simulink model "GradientAscentTrialTesting"  (R2017b)
settings: Solver=FixedStepDiscrete  StartTime=0.0  StopTime=60  FixedStep=Ts  RelTol=1e-3
PreLoadFcn:
  | ROSconfig
  | wptsSignalSetup
InitFcn:
  | config_parameters
StartFcn:
  | gazeboSetup
StopFcn:
  | gazeboReset
  | goalreset
  | loadResults
model workspace (MAT data in the model file):
  goalpoints = Simulink.Signal
  goalpoints.DataType = 'auto'
  goalpoints.Dimensions = -1
  goalpoints.DimensionsMode = 'auto'
  goalpoints.Complexity = 'auto'
  goalpoints.SampleTime = -1
  goalpoints.SamplingMode = 'auto'
  goals = Simulink.Signal
  goals.DataType = 'auto'
  goals.Dimensions = -1
  goals.DimensionsMode = 'auto'
  goals.Complexity = 'auto'
  goals.SampleTime = -1
  goals.SamplingMode = 'auto'
  idx = 1
  y = Simulink.Parameter
  y.DataType = 'auto'
  y.Dimensions = [0 0]
values from neighbouring files (symbols this model uses):
  m = [m; i*(2*pi/M)]    [SensorArrangementPlots.m]    (also in sensorArrayTesting.m = [0;0;1.2566;2.5133;3.7699;5.0265])
  sensorDist = 1    [GradientAscentMetrics.m]
undefined symbols (not defined in the file or in its folder): angmax, Angular, concDetectionAccuracy, Cthresh, DiscIntNeverNeededParam, distError, dynamicPlume, hot, inc, init, initX, initY, Kd, Ki, Kp, Linear, N, Offset, PlumeD, PlumeUpdateRate, Res, sourceAccuracy, T, Ts, vmax, wgain, WindD, WindX, x_g, y_g
libraries: simulink x21, dspindex x18, dspswit3 x4, robotlib x3, sm_lib x2, nesl_utility x1, dspsnks4 x1, mobileRoboticsLib x1
(part 1 of 2)
PauseFcn:
  | gazeboPause
settings Model: OrderedModelArguments=off  Creator=ty  LastModifiedBy=ty
settings SolverCC: AlgebraicLoopSolver=LineSearch
settings DataIOCC: ExternalInput=[r, b]  SaveFormat=Array  SaveState=on  InspectSignalLogs=on  StateSaveName=wpts
settings SimMechanicsCC: VisOnUpdateDiagram=on  VisDuringSimulation=on  DefaultBodyColor=[.877 0 0]
settings ExplorerConfigSet: SimMechanicsOpenEditorOnUpdate=off  InternalSimMechanicsExplorerSettings="<ExplorerConfiguration><canonicalview>default</canonicalview><AnimationSetting><BasePlaybackSpeed>1.0</BasePlaybackSpeed><PlaybackSpeedFactor>4.0</PlaybackSpeedFactor></AnimationSetting><TilePanel><TileInfo><Tiles Columns=\"2\" Count=\"4\" Rows=\"2\"><Column Weight=\"0.5\"/><Column Weight=\"0.5\"/><Row Weight=\"0.5\"/><Row Weight=\"0.5\"/><Tile Height=\"1\" Width=\"1\" X=\"0\" Y=\"0\"/><Tile Height=\"1\" Width=\"1\" X=\"0\" Y=\"1\"/><Tile Height=\"1\" Width=\"1\" X=\"1\" Y=\"0\"/><Tile Height=\"1\" Width=\"1\" X=\"1\" Y=\"1\"/></Tiles></TileInfo><SceneInfo><SceneViewer><BGColor><R>0.60000002384185791</R><G>0.60000002384185791</G><B>0.60000002384185791</B></BGColor><Camera><DoPerspective>off</DoPerspective><Position><X>0.523539858098702515</X><Y>-0.526832295844210763</Y><Z>1.31558763938248235</Z></Position><Center><X>0.523539858098702515</X><Y>-0.526832295844210763</Y><Z>0.315587639382482354</Z></Center><Up><X>0</X><Y>1</Y><Z>-0</Z></Up><ViewLimDist>1</ViewLimDist><YLim>8.09056691591361421</YLim><XLim>11.4549610789668002</XLim></Camera></SceneViewer><SceneViewer><BGColor><R>0.60000002384185791</R><G>0.60000002384185791</G><B>0.60000002384185791</B></BGColor><Camera><DoPerspective>off</DoPerspective><Position><X>-1.00000000034924597</X><Y>-0.123102183445061519</Y><Z>0.275798201199813964</Z></Position><Center><X>-3.49245965480804443e-10</X><Y>-0.123102183445061519</Y><Z>0.275798201199813964</Z></Center><Up><X>0</X><Y>0</Y><Z>1</Z></Up><ViewLimDist>1</ViewLimDist><YLim>3.47753295219900371</YLim><XLim>4.92363576400452985</XLim></Camera></SceneViewer><SceneViewer><BGColor><R>0.60000002384185791</R><G>0.60000002384185791</G><B>0.60000002384185791</B></BGColor><Camera><DoPerspective>off</DoPerspective><Position><X>0.692144908773628886</X><Y>-0.692774488443842151</Y><Z>0.641997243049143074</Z></Position><Center><X>0.114794639584003433</X><Y>-0.115424219254216046</Y><Z>0.0646469738595174259</Z></Center><Up><X>-0.408248290463863073</X><Y>0.408248290463863073</Y><Z>0.816496580927726145</Z></Up><ViewLimDist>1</ViewLimDist><YLim>6.0070720394774666</YLim><XLim>8.50506239252750262</XLim></Camera></SceneViewer><SceneViewer><BGColor><R>0.60000002384185791</R><G>0.60000002384185791</G><B>0.60000002384185791</B></BGColor><Camera><DoPerspective>off</DoPerspective><Position><X>0.0489598554332313918</X><Y>-0.287272213681231237</Y><Z>1.31558770067272501</Z></Position><Center><X>0.0489598554332313918</X><Y>-0.287272213681231237</Y><Z>0.315587700672725013</Z></Center><Up><X>0</X><Y>1</Y><Z>-0</Z></Up><ViewLimDist>1</ViewLimDist><YLim>2.42704539801906094</YLim><XLim>3.4363118011556999</XLim></Camera></SceneViewer></SceneInfo></TilePanel><MechEditorPanel><Cameras><Camera><Id>Camera1</Id><Value><Name>TopCamera1</Name><NativeCamera><PositionKeyframeSet><Keyframe><Time>+0.0000000000000000e+00</Time><Value><X>+2.1442706964244174e-01</X><Y>+2.3082412087368320e-01</Y><Z>+8.5801428178680403e+00</Z></Value></Keyframe></PositionKeyframeSet><CenterKeyframeSet><Keyframe><Time>+0.0000000000000000e+00</Time><Value><X>+1.7666087274208450e-01</X><Y>+1.6219238056249624e-01</Y><Z>+3.9566976367888529e-01</Z></Value></Keyframe></CenterKeyframeSet><UpVectorKeyframeSet><Keyframe><Time>+0.0000000000000000e+00</Time><Value><X>-1.4536948631457236e-02</X><Y>+9.9985973958876295e-01</Y><Z>-8.3173477730344968e-03</Z></Value></Keyframe></UpVectorKeyframeSet></NativeCamera></Value></Camera></Cameras><GfxPanelCameraMap/><VideoCreator><PlaybackSpeedRatio>1.0</PlaybackSpeedRatio><FrameRate>30</FrameRate><VideoFormat>Motion JPEG AVI</VideoFormat><FrameSize>auto</FrameSize></VideoCreator></MechEditorPanel></ExplorerConfiguration>"

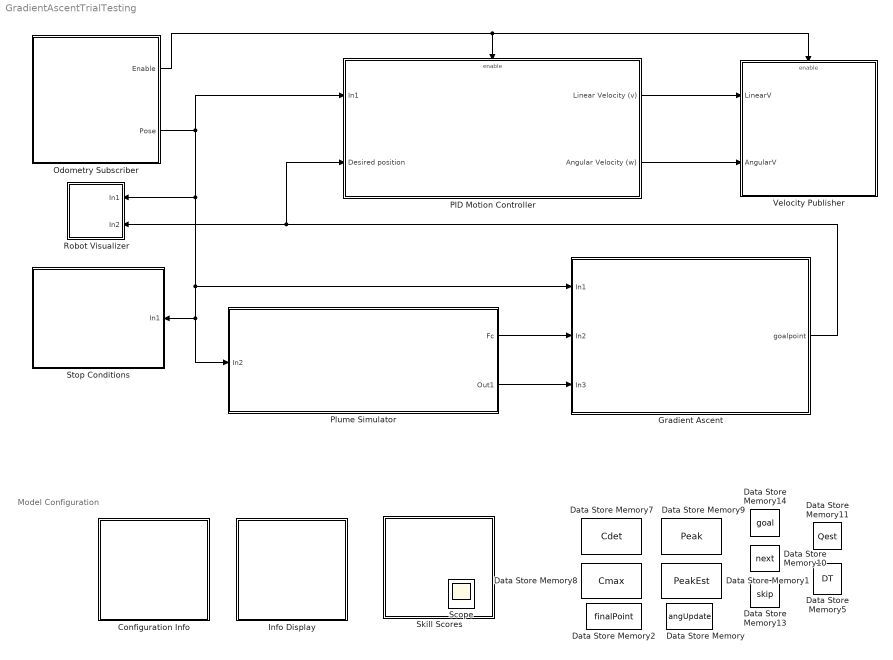
== system GradientAscentTrialTesting ==
  note: Model Configuration
  Configuration Info : Subsystem
  Data Store Memory : DataStoreMemory  DataStoreName=angUpdate  ReadBeforeWriteMsg=warning  WriteAfterWriteMsg=warning  WriteAfterReadMsg=warning  ShowAdditionalParam=off
  Data Store Memory1 : DataStoreMemory  DataStoreName=PeakEst  ReadBeforeWriteMsg=warning  WriteAfterWriteMsg=warning  WriteAfterReadMsg=warning  InitialValue=[(initX) (initY)]  VectorParams1D=off  ShowAdditionalParam=off
  Data Store Memory10 : DataStoreMemory  DataStoreName=next  ReadBeforeWriteMsg=warning  WriteAfterWriteMsg=warning  WriteAfterReadMsg=warning  ShowAdditionalParam=off
  Data Store Memory11 : DataStoreMemory  DataStoreName=Qest  ReadBeforeWriteMsg=warning  WriteAfterWriteMsg=warning  WriteAfterReadMsg=warning  ShowAdditionalParam=off
  Data Store Memory13 : DataStoreMemory  DataStoreName=skip  ReadBeforeWriteMsg=warning  WriteAfterWriteMsg=warning  WriteAfterReadMsg=warning  ShowAdditionalParam=off
  Data Store Memory14 : DataStoreMemory  DataStoreName=goal  ReadBeforeWriteMsg=warning  WriteAfterWriteMsg=warning  WriteAfterReadMsg=warning  VectorParams1D=off  ShowAdditionalParam=off
  Data Store Memory2 : DataStoreMemory  DataStoreName=finalPoint  ReadBeforeWriteMsg=warning  WriteAfterWriteMsg=warning  WriteAfterReadMsg=warning  ShowAdditionalParam=off
  Data Store Memory5 : DataStoreMemory  DataStoreName=DT  ReadBeforeWriteMsg=warning  WriteAfterWriteMsg=warning  WriteAfterReadMsg=warning  InitialValue=[0]  VectorParams1D=off  ShowAdditionalParam=off
  Data Store Memory7 : DataStoreMemory  DataStoreName=Cdet  ReadBeforeWriteMsg=warning  WriteAfterWriteMsg=warning  WriteAfterReadMsg=warning  ShowAdditionalParam=off
  Data Store Memory8 : DataStoreMemory  DataStoreName=Cmax  ReadBeforeWriteMsg=warning  WriteAfterWriteMsg=warning  WriteAfterReadMsg=warning  ShowAdditionalParam=off
  Data Store Memory9 : DataStoreMemory  DataStoreName=Peak  ReadBeforeWriteMsg=warning  WriteAfterWriteMsg=warning  WriteAfterReadMsg=warning  InitialValue=[x_g,y_g]  ShowAdditionalParam=off
  Gradient Ascent : Subsystem  mask{sensorDist=.5, mag=2}
      mask prompts: sensorDist "Sensor Distance"; mag "Update Magnitude"
  Info Display : Subsystem
  Odometry Subscriber : Subsystem
  PID Motion Controller : Subsystem
  Plume Simulator : Subsystem
  Robot Visualizer : Subsystem
  Skill Scores : Subsystem
  Stop Conditions : Subsystem
  Velocity Publisher : Subsystem
  Scope : Scope
  wires:
  Odometry Subscriber/1(Enable) -> Velocity Publisher/Enable, PID Motion Controller/Enable
  Odometry Subscriber/2(Pose) -> Plume Simulator/1(In2), Stop Conditions/1(In1), Gradient Ascent/1(In1), Robot Visualizer/1(In1), PID Motion Controller/1(In1)
  PID Motion Controller/1(Linear Velocity (v)) -> Velocity Publisher/1(LinearV)
  PID Motion Controller/2(Angular Velocity (w)) -> Velocity Publisher/2(AngularV)
  Gradient Ascent/1(goalpoint) -> PID Motion Controller/2(Desired position), Robot Visualizer/2(In2)
  Plume Simulator/1(Fc) -> Gradient Ascent/2(In2)
  Plume Simulator/2(Out1) -> Gradient Ascent/3(In3)

== system GradientAscentTrialTesting/Configuration Info ==
  note: Nodes :
      | Publishers:
      | /sim_p3at/cmd_vel
      | /toggle_led
      | Subscribers:
      | /sim_p3at/odom
      | Messages:
      | geometry_msgs/Twist
      | std_msgs/Empty
  note: Startup Programs :
      | roscore
      | roslaunch nre_p3at p3at.gazebo.launch (starts Gazebo and /sim_p3at Nodes)
      | Arduino: ledtest3.ino
      | rosrun rosserial_python serial_node.py /dev/ttyACM0
      | MATLAB: (Simulink project)
  note: SS Parameters :
      | Expansion Constant: 2
  note: Plume Parameters :
      |
      | Diffusion constant (m2/s): c_diff = .8
      |
      | Advection velocity values (m/s): ux = 0 uy = 0 uz = 0.2
      |
      | Simulation Time (seconds): T = 10
      |
      | Domain dimensions (meters): L = 50 B = 50 H = 5
  "Counter " : Subsystem  Commented=on
  Floating Scope : Scope  Commented=on
      settings: Floating=on
  MechanismConfiguration : sm_lib/Utilities/Mechanism Configuration  UniformGravity=Constant  GravityVector=[0 0 -9.80665]  GravityUnits=m/s^2  LinearizationDelta=0.01
  Solver Configuration : nesl_utility/Solver Configuration  PhysicalDomain=network_engine_domain  SubClassName=solver  LeftPortType=input  RightPortType=generic  Accelerate=off  Tones=[]  Harmonics=[]  SimulateNoise=off  Profile=off  UseLocalSampling=off  EnableSwitchedLinearOptims=on  FrequencyDomain=off  UseCCode=off  RelTol=0.001  AbsTol=1e-06  MinStep=1e-09  ToWorkspace=off  RevertToSquareIcSolve=off  NumHomotopyIterations=100  PhasorMode=off  PhasorModeNumHarmonics=1  DoDC=on  ResidualTolerance=1e-09  UseLocalSolver=on  LocalSolverChoice=NE_BACKWARD_EULER_ADVANCER  LocalSolverSampleTime=Ts  DoFixedCost=on  MaxNonlinIter=3  MaxModeIter=2  LinearAlgebra=Sparse  DelaysMemoryBudget=1024  AutomaticFiltering=on  FilteringTimeConstant=0.01
  World : sm_lib/Frames and Transforms/World Frame
  connections:
  MechanismConfiguration/RConn1 -- World/RConn1 -- Solver Configuration/RConn1

== system GradientAscentTrialTesting/Gradient Ascent ==
  In1 : Inport
  In2 : Inport  Port=2
  In3 : Inport  Port=3
  Constant : Constant  Value=sensorDist
  Constant1 : Constant  Value=N
  Data Store Read : DataStoreRead  DataStoreName=next
  Data Store Write : DataStoreWrite  DataStoreName=angUpdate
  Detect Change : simulink/Logic and Bit Operations/Detect Change  vinit=1.514  OutDataTypeStr=boolean
  Display : Display
  GradAscent : MATLAB Function  TreatAsAtomicUnit=on
  Subsystem1 : Subsystem
  goalpoint : Outport
  wires:
  In1/1 -> Subsystem1/1(pose)
  In2/1 -> GradAscent/1(C)
  In3/1 -> GradAscent/2(n)
  GradAscent/1(ang) -> Detect Change/1, Display/1, Subsystem1/3(ang)
  Subsystem1/1(goal) -> goalpoint/1
  Data Store Read/1 -> Subsystem1/2(next)
  Constant/1 -> GradAscent/4(r)
  Constant1/1 -> GradAscent/3(N)
  Detect Change/1 -> Data Store Write/1

== system GradientAscentTrialTesting/Info Display ==
  Clock : Clock
      settings: Decimation=2
  Data Store Read : DataStoreRead  DataStoreName=PeakEst
  Data Store Read1 : DataStoreRead  DataStoreName=Peak
  Data Store Read2 : DataStoreRead  DataStoreName=Cmax
  Data Store Read3 : DataStoreRead  DataStoreName=Cdet
  Data Store Read4 : DataStoreRead  DataStoreName=Qest
  Detected Concentration Levels : Subsystem  DialogController=hmiCreateDDGDialog  IsWebBlock=on  mask(MWDashboardBlock){webBlockId=6b377d99-0008-4121-aea7-73876731bd10, webBlockType=sdiscope, ShowInitialText=off, HMISrcModelName=GradientAscentTrialTesting}
      mask prompts: webBlockId "WebBlock Id"; webBlockType "WebBlock Type"; HMISrcModelName "Source Model"
      mask help: SimulinkHMI:dialogs:HMIScopeDialogDesc
      mask Help: helpview([docroot '/mapfiles/simulink.map'], 'hmi_scope')
      mask Display:
      | if strcmp(get_param(bdroot(gcb),'BlockDiagramType'), 'library')
      |     image([(matlabroot) '/toolbox/simulink/hmi/icons/DashboardScope.png']);
      | end
  Display{,1..5} (6 alike) : Display
  Localization Error : Subsystem  DialogController=hmiCreateDDGDialog  IsWebBlock=on  mask(MWDashboardBlock){webBlockId=d5e779f4-6058-4c24-8153-4ecbd3312a81, webBlockType=sdiscope, ShowInitialText=on, HMISrcModelName=GradientAscentTrialTesting}
      mask prompts: webBlockId "WebBlock Id"; webBlockType "WebBlock Type"; HMISrcModelName "Source Model"
      mask help: SimulinkHMI:dialogs:HMIScopeDialogDesc
      mask Help: helpview([docroot '/mapfiles/simulink.map'], 'hmi_scope')
      mask Display:
      | if strcmp(get_param(bdroot(gcb),'BlockDiagramType'), 'library')
      |     image([(matlabroot) '/toolbox/simulink/hmi/icons/DashboardScope.png']);
      | end
  To Workspace : ToWorkspace  VariableName=Tm  SampleTime=-1
  wires:
  Data Store Read1/1 -> Display/1
  Data Store Read/1 -> Display4/1
  Data Store Read4/1 -> Display3/1
  Data Store Read2/1 -> Display2/1
  Clock/1 -> To Workspace/1, Display1/1
  Data Store Read3/1 -> Display5/1

== system GradientAscentTrialTesting/Odometry Subscriber ==
  Odom Conversion : Subsystem
  Subscribe1 : robotlib/Subscribe  SourceLibraryInfo=This block requires Robotics System Toolbox  topicSource=Select from ROS network  topic=/sim_p3at/odom  messageType=nav_msgs/Odometry  sampleTime=-1  messageQueueLength=51
      settings: SourceProductBaseCode=RO
  Enable : Outport
  Pose : Outport  Port=2
  wires:
  Subscribe1/1 -> Enable/1
  Subscribe1/2 -> Odom Conversion/1(In1)
  Odom Conversion/1(pose) -> Pose/1

== system GradientAscentTrialTesting/PID Motion Controller ==
  In1 : Inport
  Desired position : Inport  Port=2
  Enable : EnablePort
  Constant3 : Constant  Value=0
  Demux : Demux  Outputs=3
  PID Calculations : Subsystem  mask{distThresh=0.5}
      mask prompts: distThresh "Distance Threshold"
  Switch1 : Switch  Criteria=u2 ~= 0
  Linear Velocity (v) : Outport
  Angular Velocity (w) : Outport  Port=2
  wires:
  Switch1/1 -> Angular Velocity (w)/1
  Constant3/1 -> Switch1/1
  Desired position/1 -> PID Calculations/1(SP)  "SP"
  Demux/1 -> PID Calculations/3(x)
  Demux/2 -> PID Calculations/2(y)
  Demux/3 -> PID Calculations/4(theta)
  PID Calculations/1(v) -> Linear Velocity (v)/1
  PID Calculations/3(w) -> Switch1/3
  In1/1 -> Demux/1
  PID Calculations/2(next) -> Switch1/2

== system GradientAscentTrialTesting/Plume Simulator ==
  In2 : Inport
  Plume Model Data Simulator : Subsystem
  Fc : Outport
  Out1 : Outport  Port=2
  wires:
  In2/1 -> Plume Model Data Simulator/1(In2)
  Plume Model Data Simulator/1(C) -> Fc/1
  Plume Model Data Simulator/2(n) -> Out1/1

== system GradientAscentTrialTesting/Robot Visualizer ==
  In1 : Inport
  In2 : Inport  Port=2
  Data Store Write : DataStoreWrite  DataStoreName=PeakEst
  Robot Visualizer : mobileRoboticsLib/Environments/Robot Visualizer  Priority=99  robotRadius=.34  mapName=gasMap  showTrajectory=on  hasWaypoints=on  hasLidar=off  sensorOffset=[ 0 0 ]  scanAngles=0  hasObjDetector=off  objDetectorOffset=[ 0,0 ]  objDetectorAngle=0  objDetectorFOV=0  objDetectorMaxRange=0  objectColors=[1,0,0;0,1,0;0,0,1]  objectMarkers='s'
  To Workspace : ToWorkspace  VariableName=goalpoints  SampleTime=-1
      settings: Save2DSignal=2-D array (concatenate along first dimension)
  wires:
  In1/1 -> Robot Visualizer/1  "pose"
  In2/1 -> To Workspace/1, Data Store Write/1, Robot Visualizer/2  "goalpoints"

== system GradientAscentTrialTesting/Skill Scores ==
  Location Estimate (SL) : Subsystem
  Source Estimate (SQ) : Subsystem

== system GradientAscentTrialTesting/Stop Conditions ==
  In1 : Inport
  Compare To Constant : simulink/Logic and Bit Operations/Compare To Constant  relop=>  const=concDetectionAccuracy  OutDataTypeStr=boolean
  Constant : Constant  Value=0
  Constant1 : Constant
  Counter : dspswit3/Counter  Direction=Up  CountEvent=Rising edge  CounterSize=User defined  MaxCount=255  InitialCount=0  Output=Count  HitValue=32  ResetInput=off  SamplesPerFrame=1  Ts=1  CntDtype=double  HitDtype=Logical
  Data Store Read1 : DataStoreRead  DataStoreName=Cmax
  Data Store Read3 : DataStoreRead  DataStoreName=Qest
  Data Store Read4 : DataStoreRead  DataStoreName=Peak
  Data Store Read5 : DataStoreRead  DataStoreName=PeakEst
  Data Store Read6 : DataStoreRead  DataStoreName=Peak
  Data Store Write : DataStoreWrite  DataStoreName=finalPoint
  Demux : Demux  Outputs=3
  Distance Threshold1 : simulink/Logic and Bit Operations/Compare To Constant  relop=<=  const=sourceAccuracy  OutDataTypeStr=boolean
  Distance Threshold2 : simulink/Logic and Bit Operations/Compare To Constant  relop=<=  const=.5  OutDataTypeStr=boolean
  Distance1 : Fcn  Expr=sqrt(u(1)^2+u(2)^2)
  Distance2 : Fcn  Expr=sqrt(u(1)^2+u(2)^2)
  Divide1 : Product  Inputs=*/
  Logical Operator1 : Logic  Operator=OR  AllPortsSameDT=off  OutDataTypeStr=boolean
  Mux : Mux  Inputs=2
  Stop Simulation : Stop
  Subtract1 : Sum  Inputs=+-
  Subtract2 : Sum  Inputs=+-
  Switch1 : Switch  Criteria=u2 > Threshold
  Terminator : Terminator
  wires:
  Logical Operator1/1 -> Counter/1
  Compare To Constant/1 -> Logical Operator1/2
  Data Store Read3/1 -> Divide1/1
  Data Store Read5/1 -> Subtract1/1
  Subtract1/1 -> Distance1/1
  Distance Threshold1/1 -> Logical Operator1/1
  Data Store Read4/1 -> Subtract1/2
  Data Store Read1/1 -> Divide1/2
  Distance1/1 -> Distance Threshold1/1
  Divide1/1 -> Compare To Constant/1
  Data Store Read6/1 -> Subtract2/1
  Subtract2/1 -> Distance2/1
  Distance2/1 -> Distance Threshold2/1
  Distance Threshold2/1 -> Stop Simulation/1
  Constant1/1 -> Switch1/1
  Constant/1 -> Switch1/3
  Counter/1 -> Switch1/2
  Switch1/1 -> Data Store Write/1
  In1/1 -> Demux/1
  Demux/1 -> Mux/1
  Demux/2 -> Mux/2
  Mux/1 -> Subtract2/2
  Demux/3 -> Terminator/1

== system GradientAscentTrialTesting/Velocity Publisher ==
  LinearV : Inport
  AngularV : Inport  Port=2
  Enable : EnablePort
  Blank Message : robotlib/Blank Message  SourceLibraryInfo=This block requires Robotics System Toolbox  messageType=geometry_msgs/Twist  SampleTime=-1
      settings: SourceProductBaseCode=RO
  Bus Assignment : BusAssignment  DialogController=Simulink.DDGSource_BusAssignment  AssignedSignals=Linear.X,Angular.Z
  Publish1 : robotlib/Publish  SourceLibraryInfo=This block requires Robotics System Toolbox  topicSource=Select from ROS network  topic=/sim_p3at/cmd_vel  messageType=geometry_msgs/Twist  messageQueueLength=105
      settings: SourceProductBaseCode=RO
  wires:
  AngularV/1 -> Bus Assignment/3
  Bus Assignment/1 -> Publish1/1
  LinearV/1 -> Bus Assignment/2
  Blank Message/1 -> Bus Assignment/1

== system GradientAscentTrialTesting/Configuration Info/Counter  ==
  In1 : Inport
  Counter : dspswit3/Counter  Direction=Up  CountEvent=Non-zero sample  CounterSize=User defined  MaxCount=255  InitialCount=0  Output=Count  HitValue=32  ResetInput=off  SamplesPerFrame=1  Ts=1  CntDtype=single  HitDtype=Logical
  Counter1 : dspswit3/Counter  Direction=Up  CountEvent=Rising edge  CounterSize=User defined  MaxCount=255  InitialCount=0  Output=Count  HitValue=32  ResetInput=off  SamplesPerFrame=1  Ts=1  CntDtype=double  HitDtype=Logical
  Detect Increase : simulink/Logic and Bit Operations/Detect Increase  vinit=0.0  OutDataTypeStr=boolean
  Out1 : Outport
  wires:
  In1/1 -> Counter/1
  Counter/1 -> Detect Increase/1
  Detect Increase/1 -> Counter1/1
  Counter1/1 -> Out1/1

== system GradientAscentTrialTesting/Gradient Ascent/Subsystem1 ==
  pose : Inport
  next : Inport  Port=2
  ang : Inport  Port=3
  Goal Update : Subsystem
  Goal Update Conditions : Subsystem
  Initialize Goal : Subsystem
  Skip Conditions : Subsystem
  goal : Outport
  wires:
  pose/1 -> Goal Update/1(In2)
  ang/1 -> Goal Update/2(In3)
  Goal Update Conditions/1(Out1) -> Goal Update/Enable
  next/1 -> Skip Conditions/1(In1)
  Initialize Goal/1(goal) -> Goal Update Conditions/1(In1), goal/1
  Goal Update/1(Out2) -> Initialize Goal/1(In1)

== system GradientAscentTrialTesting/Info Display/Detected Concentration Levels ==

== system GradientAscentTrialTesting/Info Display/Localization Error ==

== system GradientAscentTrialTesting/Odometry Subscriber/Odom Conversion ==
  In1 : Inport
  Bus Selector3 : BusSelector  OutputSignals=Pose.Pose.Position.X,Pose.Pose.Position.Y,Pose.Pose.Orientation.X,Pose.Pose.Orientation.Y,Pose.Pose.Orientation.Z,Pose.Pose.Orientation.W
  Conversion : MATLAB Function  TreatAsAtomicUnit=on
  Mux : Mux  Inputs=3
  pose : Outport
  wires:
  In1/1 -> Bus Selector3/1
  Bus Selector3/3 -> Conversion/1(x)  "<X>"
  Bus Selector3/4 -> Conversion/2(y)  "<Y>"
  Bus Selector3/5 -> Conversion/3(z)  "<Z>"
  Bus Selector3/6 -> Conversion/4(w)  "<W>"
  Bus Selector3/2 -> Mux/2  "<Y>"
  Bus Selector3/1 -> Mux/1  "<X>"
  Mux/1 -> pose/1  "pose"
  Conversion/1(yaw) -> Mux/3

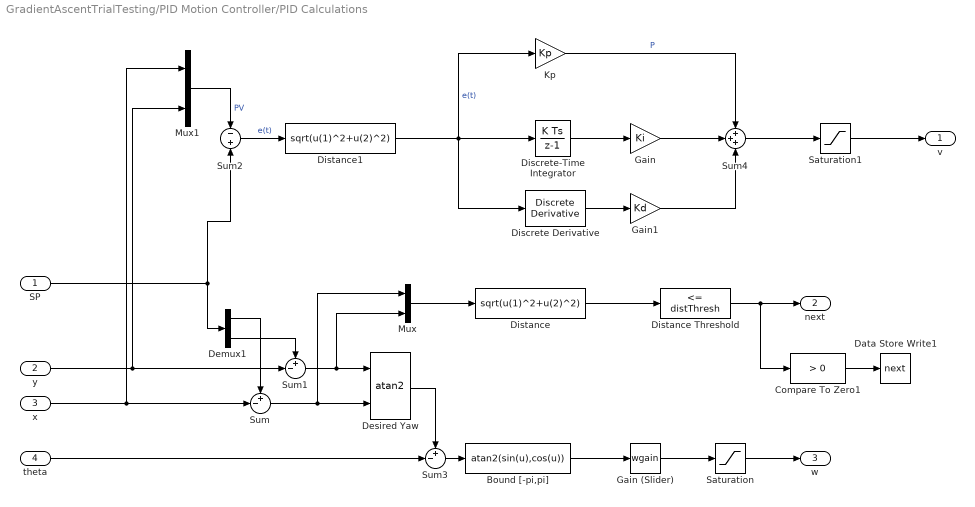
== system GradientAscentTrialTesting/PID Motion Controller/PID Calculations ==
  SP : Inport
  y : Inport  Port=2
  x : Inport  Port=3
  theta : Inport  Port=4
  Bound [-pi,pi] : Fcn  Expr=atan2(sin(u),cos(u))
  Compare To Zero1 : simulink/Logic and Bit Operations/Compare To Zero  relop=>  OutDataTypeStr=boolean
  Data Store Write1 : DataStoreWrite  DataStoreName=next
  Demux1 : Demux  Outputs=2
  Desired Yaw : Trigonometry  Operator=atan2
  Discrete Derivative : simulink/Discrete/Discrete Derivative  gainval=1  ICPrevScaledInput=0.0  OutMin=[]  OutMax=[]  OutDataType=fixdt(1, 16)  OutScaling=2^-10  DoSatur=off
  Discrete-Time Integrator : DiscreteIntegrator  gainval=1  InitialConditionSetting=State (most efficient)  SampleTime=-1  ICPrevOutput=DiscIntNeverNeededParam  ICPrevScaledInput=DiscIntNeverNeededParam
  Distance : Fcn  Expr=sqrt(u(1)^2+u(2)^2)
  Distance Threshold : simulink/Logic and Bit Operations/Compare To Constant  relop=<=  const=distThresh  OutDataTypeStr=boolean
  Distance1 : Fcn  Expr=sqrt(u(1)^2+u(2)^2)
  Gain : Gain  Gain=Ki
  Gain (Slider) : simulink/Math Operations/Slider Gain  gain=wgain  low=1  high=10
  Gain1 : Gain  Gain=Kd
  Kp : Gain  Gain=Kp
  Mux : Mux  Inputs=2
  Mux1 : Mux  Inputs=2
  Saturation : Saturate  UpperLimit=angmax  LowerLimit=-angmax
  Saturation1 : Saturate  UpperLimit=vmax  LowerLimit=-.5
  Sum : Sum  Inputs=+-|
  Sum1 : Sum  Inputs=+-|
  Sum2 : Sum  Inputs=-+
  Sum3 : Sum  Inputs=+-|
  Sum4 : Sum  Inputs=+++
  v : Outport
  next : Outport  Port=2
  w : Outport  Port=3
  wires:
  theta/1 -> Sum3/2
  Desired Yaw/1 -> Sum3/1
  Sum/1 -> Desired Yaw/2, Mux/1
  Gain (Slider)/1 -> Saturation/1
  Saturation/1 -> w/1
  Sum3/1 -> Bound [-pi,pi]/1
  Mux1/1 -> Sum2/1  "PV"
  Kp/1 -> Sum4/1  "P"
  Distance1/1 -> Kp/1, Discrete-Time Integrator/1, Discrete Derivative/1  "e(t)"
  Discrete-Time Integrator/1 -> Gain/1
  Demux1/1 -> Sum/1
  Demux1/2 -> Sum1/1
  Sum1/1 -> Desired Yaw/1, Mux/2
  SP/1 -> Demux1/1, Sum2/2
  y/1 -> Mux1/2, Sum1/2
  x/1 -> Mux1/1, Sum/2
  Distance/1 -> Distance Threshold/1
  Mux/1 -> Distance/1
  Bound [-pi,pi]/1 -> Gain (Slider)/1
  Sum2/1 -> Distance1/1  "e(t)"
  Gain/1 -> Sum4/2
  Sum4/1 -> Saturation1/1
  Discrete Derivative/1 -> Gain1/1
  Gain1/1 -> Sum4/3
  Saturation1/1 -> v/1
  Distance Threshold/1 -> Compare To Zero1/1, next/1
  Compare To Zero1/1 -> Data Store Write1/1

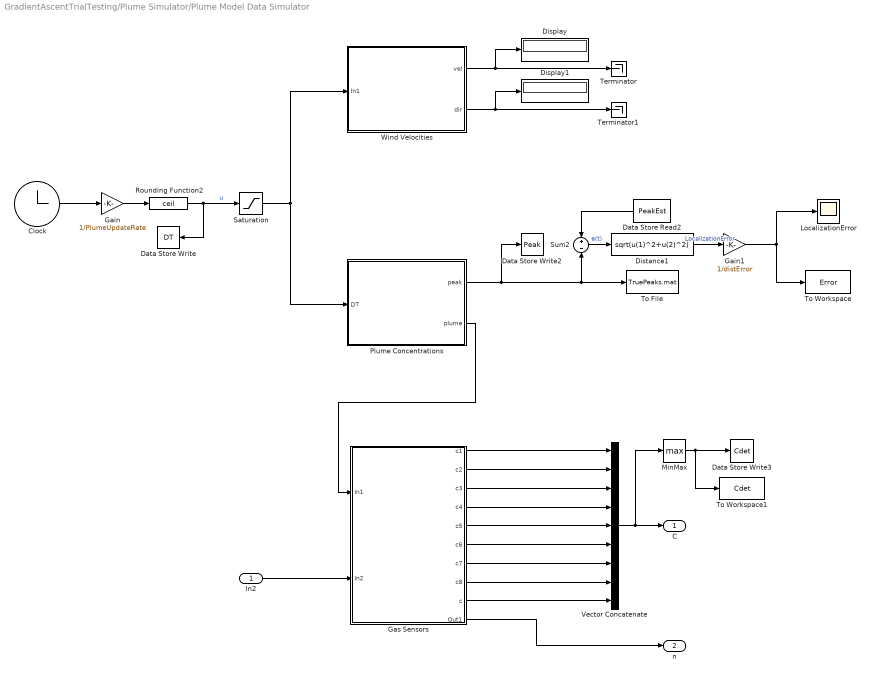
== system GradientAscentTrialTesting/Plume Simulator/Plume Model Data Simulator ==
  In2 : Inport
  Clock : Clock
      settings: Decimation=3
  Data Store Read2 : DataStoreRead  DataStoreName=PeakEst
  Data Store Write : DataStoreWrite  DataStoreName=DT
  Data Store Write2 : DataStoreWrite  DataStoreName=Peak
  Data Store Write3 : DataStoreWrite  DataStoreName=Cdet
  Display : Display
  Display1 : Display
  Distance1 : Fcn  Expr=sqrt(u(1)^2+u(2)^2)
  Gain : Gain  Gain=1/PlumeUpdateRate
  Gain1 : Gain  Gain=1/distError
  Gas Sensors : Subsystem
  LocalizationError : Scope
  MinMax : MinMax  Function=max
  Plume Concentrations : Subsystem
  Rounding Function2 : Rounding  Operator=ceil
  Saturation : Saturate  UpperLimit=T/Ts  LowerLimit=1
  Sum2 : Sum  Inputs=+-
  Terminator : Terminator
  Terminator1 : Terminator
  To File : ToFile  Filename=TruePeaks.mat  MatrixName=ActualPeaks
      settings: Decimation=2
  To Workspace : ToWorkspace  VariableName=Error  SaveFormat=Timeseries  SampleTime=-1
  To Workspace1 : ToWorkspace  VariableName=Cdet  SaveFormat=Timeseries  SampleTime=-1
  Vector Concatenate : Concatenate  NumInputs=9
  Wind Velocities : Subsystem
  C : Outport
  n : Outport  Port=2
  wires:
  Clock/1 -> Gain/1
  Rounding Function2/1 -> Saturation/1, Data Store Write/1  "u"
  In2/1 -> Gas Sensors/2(In2)
  Gain/1 -> Rounding Function2/1
  Sum2/1 -> Distance1/1  "e(t)"
  Data Store Read2/1 -> Sum2/1
  Distance1/1 -> Gain1/1  "LocalizationError"
  Plume Concentrations/1(peak) -> Data Store Write2/1, To File/1, Sum2/2
  Saturation/1 -> Wind Velocities/1(In1), Plume Concentrations/1(DT)
  Wind Velocities/1(vel) -> Terminator/1, Display/1
  Wind Velocities/2(dir) -> Terminator1/1, Display1/1
  Plume Concentrations/2(plume) -> Gas Sensors/1(In1)
  Gas Sensors/1(c1) -> Vector Concatenate/1
  Gas Sensors/2(c2) -> Vector Concatenate/2
  Gas Sensors/3(c3) -> Vector Concatenate/3
  Gas Sensors/4(c4) -> Vector Concatenate/4
  Vector Concatenate/1 -> MinMax/1, C/1
  Gas Sensors/5(c5) -> Vector Concatenate/5
  Gas Sensors/6(c6) -> Vector Concatenate/6
  Gas Sensors/7(c7) -> Vector Concatenate/7
  Gas Sensors/8(c8) -> Vector Concatenate/8
  Gas Sensors/9(c) -> Vector Concatenate/9
  Gas Sensors/10(Out1) -> n/1
  MinMax/1 -> To Workspace1/1, Data Store Write3/1
  Gain1/1 -> To Workspace/1, LocalizationError/1

== system GradientAscentTrialTesting/Skill Scores/Location Estimate (SL) ==
  Data Store Read : DataStoreRead  DataStoreName=Peak
  Data Store Read2 : DataStoreRead  DataStoreName=PeakEst
  Distance : Fcn  Expr=sqrt(u(1)^2+u(2)^2)
  Distance Threshold : simulink/Logic and Bit Operations/Compare To Constant  Commented=on  relop=<=  const=sourceAccuracy  OutDataTypeStr=boolean
  Gain : Gain  Gain=1/distError
  Stop Simulation : Stop  Commented=on
  Subtract : Sum  Inputs=+-
  To Workspace1 : ToWorkspace  VariableName=ScoreL  SampleTime=-1
      settings: Save2DSignal=2-D array (concatenate along first dimension)
  wires:
  Data Store Read/1 -> Subtract/2
  Subtract/1 -> Distance/1
  Data Store Read2/1 -> Subtract/1
  Distance Threshold/1 -> Stop Simulation/1
  Distance/1 -> Gain/1, Distance Threshold/1
  Gain/1 -> To Workspace1/1

== system GradientAscentTrialTesting/Skill Scores/Source Estimate (SQ) ==
  Abs : Abs
  Data Store Read : DataStoreRead  DataStoreName=Qest
  Data Store Read1 : DataStoreRead  DataStoreName=Cmax
  Divide : Product  Inputs=*/
  Q estimate : Subsystem
  Subtract1 : Sum  Inputs=-+
  To Workspace : ToWorkspace  VariableName=ScoreQ  SampleTime=-1
  wires:
  Divide/1 -> Abs/1
  Subtract1/1 -> Divide/1
  Abs/1 -> To Workspace/1
  Data Store Read/1 -> Subtract1/1
  Data Store Read1/1 -> Divide/2, Subtract1/2

== system GradientAscentTrialTesting/Gradient Ascent/Subsystem1/Goal Update ==
  In2 : Inport
  In3 : Inport  Port=2
  Enable : EnablePort
  Constant : Constant  Value=mag
  goalUpdate : MATLAB Function  TreatAsAtomicUnit=on
  Out2 : Outport
  wires:
  In3/1 -> goalUpdate/2(ang)
  goalUpdate/1(goal) -> Out2/1
  In2/1 -> goalUpdate/1(pose)
  Constant/1 -> goalUpdate/3(mag)

== system GradientAscentTrialTesting/Gradient Ascent/Subsystem1/Goal Update Conditions ==
  In1 : Inport
  Data Store Read : DataStoreRead  DataStoreName=Peak
  Data Store Read1 : DataStoreRead  DataStoreName=angUpdate
  Data Store Read2 : DataStoreRead  DataStoreName=next
  Distance : Fcn  Expr=sqrt(u(1)^2+u(2)^2)
  Distance Threshold : simulink/Logic and Bit Operations/Compare To Constant  relop=<=  const=sourceAccuracy  OutDataTypeStr=boolean
  Logical Operator : Logic  Operator=OR  AllPortsSameDT=off  OutDataTypeStr=boolean
  Logical Operator1 : Logic  Operator=OR  AllPortsSameDT=off  OutDataTypeStr=boolean
  Subtract : Sum  Inputs=+-
  Out1 : Outport
  wires:
  In1/1 -> Subtract/1
  Subtract/1 -> Distance/1
  Distance/1 -> Distance Threshold/1
  Distance Threshold/1 -> Logical Operator/2
  Data Store Read2/1 -> Logical Operator/1
  Logical Operator/1 -> Logical Operator1/1
  Data Store Read/1 -> Subtract/2
  Data Store Read1/1 -> Logical Operator1/2
  Logical Operator1/1 -> Out1/1

== system GradientAscentTrialTesting/Gradient Ascent/Subsystem1/Initialize Goal ==
  In1 : Inport
  Constant : Constant  Value=init
  Data Store Read : DataStoreRead  DataStoreName=skip
  Data Store Read1 : DataStoreRead  DataStoreName=finalPoint
  Data Store Read2 : DataStoreRead  DataStoreName=PeakEst
  Switch : Switch  Criteria=u2 > Threshold
  Switch1 : Switch  Criteria=u2 > Threshold
  goal : Outport
  wires:
  Data Store Read/1 -> Switch/2
  In1/1 -> Switch/1
  Constant/1 -> Switch/3
  Switch/1 -> Switch1/3
  Data Store Read1/1 -> Switch1/2
  Data Store Read2/1 -> Switch1/1
  Switch1/1 -> goal/1

== system GradientAscentTrialTesting/Gradient Ascent/Subsystem1/Skip Conditions ==
  In1 : Inport
  Constant1 : Constant
  Counter : dspswit3/Counter  Direction=Up  CountEvent=Rising edge  CounterSize=User defined  MaxCount=255  InitialCount=0  Output=Count  HitValue=32  ResetInput=off  SamplesPerFrame=1  Ts=1  CntDtype=double  HitDtype=Logical
  Data Store Write4 : DataStoreWrite  DataStoreName=skip
  Ground1 : Ground
  Switch1 : Switch  Criteria=u2 > Threshold
  wires:
  Constant1/1 -> Switch1/1
  Counter/1 -> Switch1/2
  Switch1/1 -> Data Store Write4/1
  Ground1/1 -> Switch1/3
  In1/1 -> Counter/1

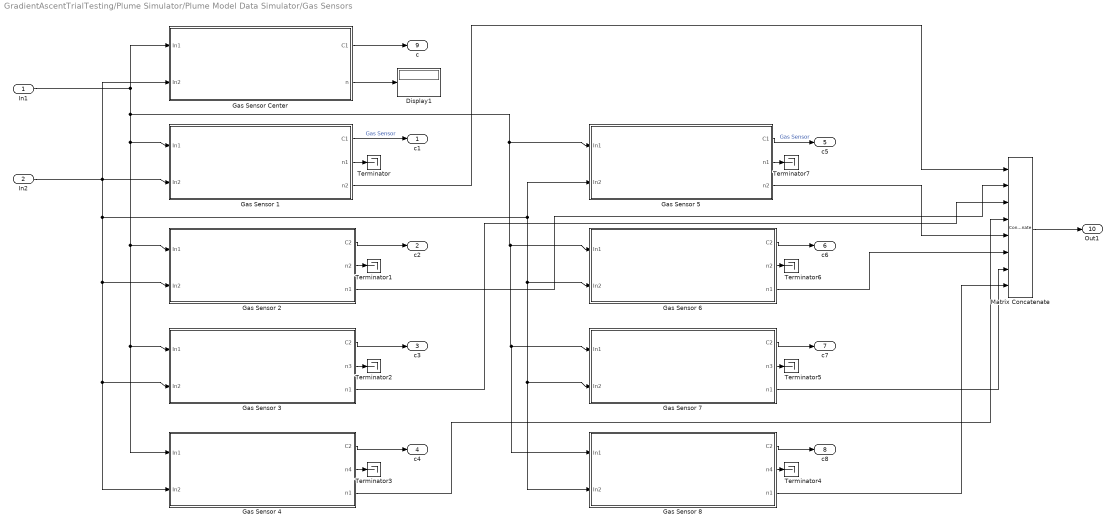
== system GradientAscentTrialTesting/Plume Simulator/Plume Model Data Simulator/Gas Sensors ==
  In1 : Inport
  In2 : Inport  Port=2
  Display1 : Display
  Gas Sensor 1 : Subsystem
  Gas Sensor 2 : Subsystem
  Gas Sensor 3 : Subsystem
  Gas Sensor 4 : Subsystem
  Gas Sensor 5 : Subsystem
  Gas Sensor 6 : Subsystem
  Gas Sensor 7 : Subsystem
  Gas Sensor 8 : Subsystem
  Gas Sensor Center : Subsystem
  Matrix Concatenate : Concatenate  NumInputs=8  Mode=Multidimensional array  ConcatenateDimension=2
  Terminator{,1..7} (8 alike) : Terminator
  c1 : Outport
  c2 : Outport  Port=2
  c3 : Outport  Port=3
  c4 : Outport  Port=4
  c5 : Outport  Port=5
  c6 : Outport  Port=6
  c7 : Outport  Port=7
  c8 : Outport  Port=8
  c : Outport  Port=9
  Out1 : Outport  Port=10
  wires:
  Gas Sensor 3/1(C2) -> c3/1
  Gas Sensor 4/1(C2) -> c4/1
  Gas Sensor 1/1(C1) -> c1/1  "Gas Sensor"
  Gas Sensor 2/1(C2) -> c2/1
  In1/1 -> Gas Sensor Center/1(In1), Gas Sensor 8/1(In1), Gas Sensor 7/1(In1), Gas Sensor 6/1(In1), Gas Sensor 5/1(In1), Gas Sensor 2/1(In1), Gas Sensor 4/1(In1), Gas Sensor 3/1(In1), Gas Sensor 1/1(In1)
  In2/1 -> Gas Sensor Center/2(In2), Gas Sensor 8/2(In2), Gas Sensor 7/2(In2), Gas Sensor 6/2(In2), Gas Sensor 5/2(In2), Gas Sensor 4/2(In2), Gas Sensor 3/2(In2), Gas Sensor 2/2(In2), Gas Sensor 1/2(In2)
  Gas Sensor Center/1(C1) -> c/1
  Gas Sensor Center/2(n) -> Display1/1
  Gas Sensor 5/1(C1) -> c5/1  "Gas Sensor"
  Gas Sensor 6/1(C2) -> c6/1
  Gas Sensor 7/1(C2) -> c7/1
  Gas Sensor 8/1(C2) -> c8/1
  Gas Sensor 1/3(n2) -> Matrix Concatenate/1
  Gas Sensor 2/3(n1) -> Matrix Concatenate/2
  Gas Sensor 3/3(n1) -> Matrix Concatenate/3
  Gas Sensor 4/3(n1) -> Matrix Concatenate/4
  Gas Sensor 5/3(n2) -> Matrix Concatenate/5
  Gas Sensor 6/3(n1) -> Matrix Concatenate/6
  Gas Sensor 7/3(n1) -> Matrix Concatenate/7
  Gas Sensor 8/3(n1) -> Matrix Concatenate/8
  Matrix Concatenate/1 -> Out1/1
  Gas Sensor 1/2(n1) -> Terminator/1
  Gas Sensor 2/2(n2) -> Terminator1/1
  Gas Sensor 3/2(n3) -> Terminator2/1
  Gas Sensor 4/2(n4) -> Terminator3/1
  Gas Sensor 8/2(n4) -> Terminator4/1
  Gas Sensor 7/2(n3) -> Terminator5/1
  Gas Sensor 6/2(n2) -> Terminator6/1
  Gas Sensor 5/2(n1) -> Terminator7/1

== system GradientAscentTrialTesting/Plume Simulator/Plume Model Data Simulator/Plume Concentrations ==
  DT : Inport
  Constant : Constant  Value=Offset
  Constant1 : Constant  Value=T/Ts
  Constant2 : Constant  Value=dynamicPlume
  Data Store Write1 : DataStoreWrite  DataStoreName=Cmax
  Dynamic Plume Concentration Data : Constant  Value=PlumeD  VectorParams1D=off  OutDataTypeStr=double  LockScale=on
  Gain1 : Gain  Gain=Res
  MATLAB Function : MATLAB Function  TreatAsAtomicUnit=on
  Matrix Viewer : dspsnks4/Matrix Viewer  Commented=on  ImageParams=off  CMapStr=hot(256)  AxisColorbar=on  AxisParams=off  AxisOrigin=Lower left corner  AxisTickMode=Auto  XTickRange=[0 1]  YTickRange=[0 1]  XLabel=X (quarter meters)  YLabel=Y (quarter meters)  ZLabel=Concentration  FigPos=[0 1750 500 400]  AxisZoom=off
      settings: SourceProductName=DSP System Toolbox  SourceProductBaseCode=DS  YMin=0  YMax=1000
  Permute Dimensions1 : PermuteDimensions
  Subtract : Sum  Inputs=+-
  Switch : Switch  Criteria=u2 > Threshold
  To Workspace3 : ToWorkspace  VariableName=Cmax  SaveFormat=Timeseries  SampleTime=-1
  peak : Outport
  plume : Outport  Port=2
  wires:
  Dynamic Plume Concentration Data/1 -> MATLAB Function/1(PlumeD)
  MATLAB Function/2(Cmax) -> To Workspace3/1, Data Store Write1/1
  Subtract/1 -> Gain1/1
  Constant/1 -> Subtract/2
  MATLAB Function/1(Plume) -> Matrix Viewer/1, Permute Dimensions1/1
  MATLAB Function/3(Peak) -> Subtract/1
  Permute Dimensions1/1 -> plume/1
  Gain1/1 -> peak/1
  DT/1 -> Switch/1
  Constant1/1 -> Switch/3
  Constant2/1 -> Switch/2
  Switch/1 -> MATLAB Function/2(u)

== system GradientAscentTrialTesting/Plume Simulator/Plume Model Data Simulator/Wind Velocities ==
  In1 : Inport
  Constant1 : Constant  Value=45
  Constant2 : Constant  Value=dynamicPlume
  Forward Wind Data : Constant  Value=WindD  VectorParams1D=off  OutDataTypeStr=double  LockScale=on
  Lateral Wind Data : Constant  Value=WindX  VectorParams1D=off  OutDataTypeStr=double  LockScale=on
  MATLAB Function : MATLAB Function  TreatAsAtomicUnit=on
  Switch : Switch  Criteria=u2 > Threshold
  vel : Outport
  dir : Outport  Port=2
  wires:
  Lateral Wind Data/1 -> MATLAB Function/1(WindX)
  In1/1 -> Switch/1
  Forward Wind Data/1 -> MATLAB Function/2(WindY)
  MATLAB Function/1(WindSpeed) -> vel/1
  MATLAB Function/2(WindDirection) -> dir/1
  Constant1/1 -> Switch/3
  Constant2/1 -> Switch/2
  Switch/1 -> MATLAB Function/3(u)

== system GradientAscentTrialTesting/Skill Scores/Source Estimate (SQ)/Q estimate ==
  Data Store Read : DataStoreRead  DataStoreName=Cdet
  Data Store Read1 : DataStoreRead  DataStoreName=Qest
  Data Store Read3 : DataStoreRead  DataStoreName=Qest
  Data Store Write2 : DataStoreWrite  DataStoreName=Qest
  Detect Increase : simulink/Logic and Bit Operations/Detect Increase  vinit=0.0  OutDataTypeStr=boolean
  Ground : Ground
  Relational Operator : RelationalOperator  OutDataTypeStr=boolean  RndMeth=Simplest
  Switch2 : Switch  Criteria=u2 > Threshold
  Switch3 : Switch  Criteria=u2 > Threshold
  To Workspace2 : ToWorkspace  VariableName=Qest  SaveFormat=Timeseries  SampleTime=-1
  wires:
  Ground/1 -> Switch2/3
  Detect Increase/1 -> Switch2/2
  Relational Operator/1 -> Switch3/2
  Switch2/1 -> Switch3/1, Relational Operator/1
  Data Store Read3/1 -> Switch3/3
  Switch3/1 -> To Workspace2/1, Data Store Write2/1  "Estimated Maximum"
  Data Store Read1/1 -> Relational Operator/2
  Data Store Read/1 -> Switch2/1, Detect Increase/1  "<Gas Sensor>"

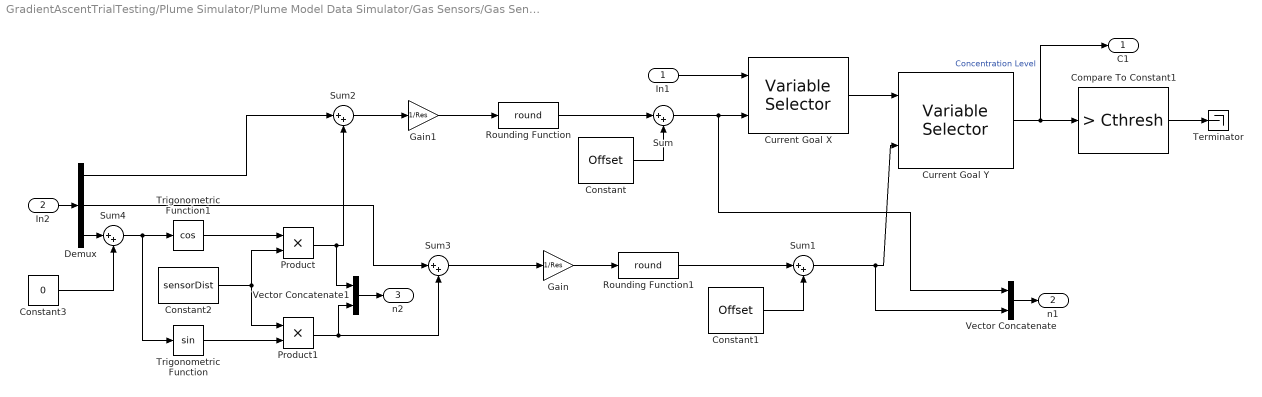
== system GradientAscentTrialTesting/Plume Simulator/Plume Model Data Simulator/Gas Sensors/Gas Sensor 1 ==
  In1 : Inport
  In2 : Inport  Port=2
  Compare To Constant1 : simulink/Logic and Bit Operations/Compare To Constant  relop=>  const=Cthresh  OutDataTypeStr=boolean
  Constant : Constant  Value=Offset
  Constant1 : Constant  Value=Offset
  Constant2 : Constant  Value=sensorDist
  Constant3 : Constant  Value=0
  Current Goal X : dspindex/Variable Selector  NumInputs=1  rowsOrCols=Rows  IdxMode=Variable  Elements=[1 3]  ZerOneIdxMode=One-based  errmode=Clip Index  FillMode=off  FillValues=0
  Current Goal Y : dspindex/Variable Selector  NumInputs=1  rowsOrCols=Columns  IdxMode=Variable  Elements=[1 3]  ZerOneIdxMode=One-based  errmode=Clip Index  FillMode=off  FillValues=0
  Demux : Demux  Outputs=3
  Gain : Gain  Gain=1/Res
  Gain1 : Gain  Gain=1/Res
  Product : Product
  Product1 : Product
  Rounding Function : Rounding  Operator=round
  Rounding Function1 : Rounding  Operator=round
  Sum{,1..4} (5 alike) : Sum  Inputs=|++
  Terminator : Terminator
  Trigonometric Function : Trigonometry
  Trigonometric Function1 : Trigonometry  Operator=cos
  Vector Concatenate : Concatenate
  Vector Concatenate1 : Concatenate
  C1 : Outport
  n1 : Outport  Port=2
  n2 : Outport  Port=3
  wires:
  In1/1 -> Current Goal X/1
  Rounding Function/1 -> Sum/1
  Current Goal Y/1 -> C1/1, Compare To Constant1/1  "Concentration Level"
  Rounding Function1/1 -> Sum1/1
  Current Goal X/1 -> Current Goal Y/1
  Constant/1 -> Sum/2
  Compare To Constant1/1 -> Terminator/1
  Constant1/1 -> Sum1/2
  Sum/1 -> Vector Concatenate/1, Current Goal X/2
  Sum1/1 -> Vector Concatenate/2, Current Goal Y/2
  Gain1/1 -> Rounding Function/1
  Gain/1 -> Rounding Function1/1
  Sum2/1 -> Gain1/1
  Sum3/1 -> Gain/1
  In2/1 -> Demux/1
  Demux/1 -> Sum2/1
  Demux/2 -> Sum3/1
  Trigonometric Function1/1 -> Product/1
  Constant2/1 -> Product1/1, Product/2
  Trigonometric Function/1 -> Product1/2
  Product/1 -> Vector Concatenate1/1, Sum2/2
  Product1/1 -> Vector Concatenate1/2, Sum3/2
  Vector Concatenate/1 -> n1/1
  Demux/3 -> Sum4/1
  Sum4/1 -> Trigonometric Function/1, Trigonometric Function1/1
  Constant3/1 -> Sum4/2
  Vector Concatenate1/1 -> n2/1

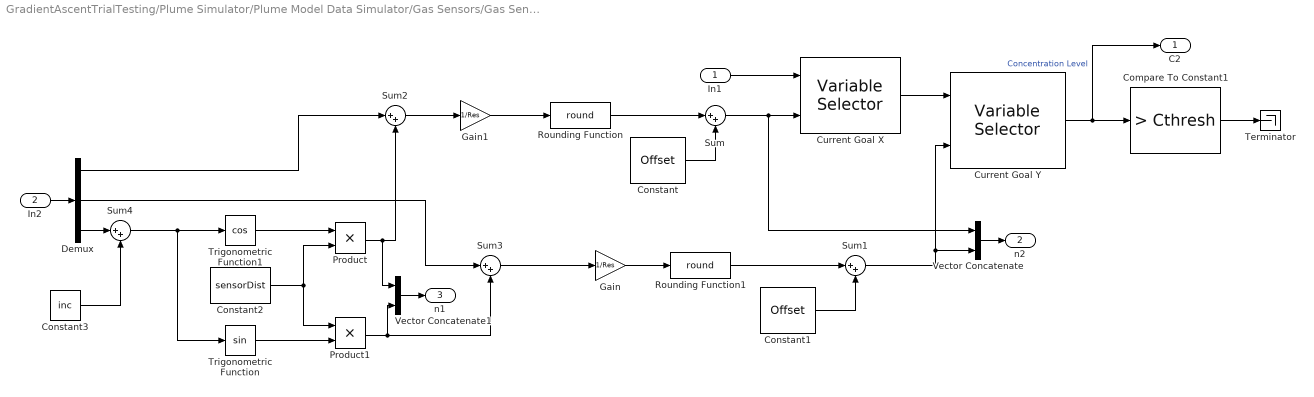
== system GradientAscentTrialTesting/Plume Simulator/Plume Model Data Simulator/Gas Sensors/Gas Sensor 2 ==
  In1 : Inport
  In2 : Inport  Port=2
  Compare To Constant1 : simulink/Logic and Bit Operations/Compare To Constant  relop=>  const=Cthresh  OutDataTypeStr=boolean
  Constant : Constant  Value=Offset
  Constant1 : Constant  Value=Offset
  Constant2 : Constant  Value=sensorDist
  Constant3 : Constant  Value=inc
  Current Goal X : dspindex/Variable Selector  NumInputs=1  rowsOrCols=Rows  IdxMode=Variable  Elements=[1 3]  ZerOneIdxMode=One-based  errmode=Clip Index  FillMode=off  FillValues=0
  Current Goal Y : dspindex/Variable Selector  NumInputs=1  rowsOrCols=Columns  IdxMode=Variable  Elements=[1 3]  ZerOneIdxMode=One-based  errmode=Clip Index  FillMode=off  FillValues=0
  Demux : Demux  Outputs=3
  Gain : Gain  Gain=1/Res
  Gain1 : Gain  Gain=1/Res
  Product : Product
  Product1 : Product
  Rounding Function : Rounding  Operator=round
  Rounding Function1 : Rounding  Operator=round
  Sum{,1..4} (5 alike) : Sum  Inputs=|++
  Terminator : Terminator
  Trigonometric Function : Trigonometry
  Trigonometric Function1 : Trigonometry  Operator=cos
  Vector Concatenate : Concatenate
  Vector Concatenate1 : Concatenate
  C2 : Outport
  n2 : Outport  Port=2
  n1 : Outport  Port=3
  wires:
  In1/1 -> Current Goal X/1
  Rounding Function/1 -> Sum/1
  Current Goal Y/1 -> C2/1, Compare To Constant1/1  "Concentration Level"
  Rounding Function1/1 -> Sum1/1
  Current Goal X/1 -> Current Goal Y/1
  Constant/1 -> Sum/2
  Compare To Constant1/1 -> Terminator/1
  Constant1/1 -> Sum1/2
  Sum/1 -> Vector Concatenate/1, Current Goal X/2
  Sum1/1 -> Vector Concatenate/2, Current Goal Y/2
  Gain1/1 -> Rounding Function/1
  Gain/1 -> Rounding Function1/1
  Sum2/1 -> Gain1/1
  Sum3/1 -> Gain/1
  In2/1 -> Demux/1
  Demux/1 -> Sum2/1
  Demux/2 -> Sum3/1
  Trigonometric Function1/1 -> Product/1
  Constant2/1 -> Product1/1, Product/2
  Trigonometric Function/1 -> Product1/2
  Product/1 -> Vector Concatenate1/1, Sum2/2
  Product1/1 -> Vector Concatenate1/2, Sum3/2
  Demux/3 -> Sum4/1
  Sum4/1 -> Trigonometric Function/1, Trigonometric Function1/1
  Constant3/1 -> Sum4/2
  Vector Concatenate/1 -> n2/1
  Vector Concatenate1/1 -> n1/1

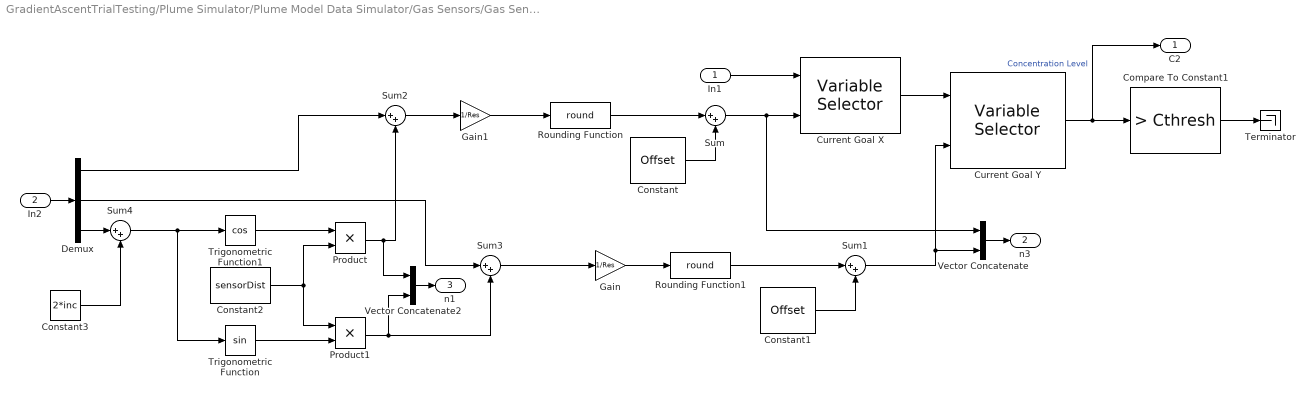
== system GradientAscentTrialTesting/Plume Simulator/Plume Model Data Simulator/Gas Sensors/Gas Sensor 3 ==
  In1 : Inport
  In2 : Inport  Port=2
  Compare To Constant1 : simulink/Logic and Bit Operations/Compare To Constant  relop=>  const=Cthresh  OutDataTypeStr=boolean
  Constant : Constant  Value=Offset
  Constant1 : Constant  Value=Offset
  Constant2 : Constant  Value=sensorDist
  Constant3 : Constant  Value=2*inc
  Current Goal X : dspindex/Variable Selector  NumInputs=1  rowsOrCols=Rows  IdxMode=Variable  Elements=[1 3]  ZerOneIdxMode=One-based  errmode=Clip Index  FillMode=off  FillValues=0
  Current Goal Y : dspindex/Variable Selector  NumInputs=1  rowsOrCols=Columns  IdxMode=Variable  Elements=[1 3]  ZerOneIdxMode=One-based  errmode=Clip Index  FillMode=off  FillValues=0
  Demux : Demux  Outputs=3
  Gain : Gain  Gain=1/Res
  Gain1 : Gain  Gain=1/Res
  Product : Product
  Product1 : Product
  Rounding Function : Rounding  Operator=round
  Rounding Function1 : Rounding  Operator=round
  Sum{,1..4} (5 alike) : Sum  Inputs=|++
  Terminator : Terminator
  Trigonometric Function : Trigonometry
  Trigonometric Function1 : Trigonometry  Operator=cos
  Vector Concatenate : Concatenate
  Vector Concatenate2 : Concatenate
  C2 : Outport
  n3 : Outport  Port=2
  n1 : Outport  Port=3
  wires:
  In1/1 -> Current Goal X/1
  Rounding Function/1 -> Sum/1
  Current Goal Y/1 -> C2/1, Compare To Constant1/1  "Concentration Level"
  Rounding Function1/1 -> Sum1/1
  Current Goal X/1 -> Current Goal Y/1
  Constant/1 -> Sum/2
  Compare To Constant1/1 -> Terminator/1
  Constant1/1 -> Sum1/2
  Sum/1 -> Vector Concatenate/1, Current Goal X/2
  Sum1/1 -> Vector Concatenate/2, Current Goal Y/2
  Gain1/1 -> Rounding Function/1
  Gain/1 -> Rounding Function1/1
  Sum2/1 -> Gain1/1
  Sum3/1 -> Gain/1
  In2/1 -> Demux/1
  Demux/1 -> Sum2/1
  Demux/2 -> Sum3/1
  Trigonometric Function1/1 -> Product/1
  Constant2/1 -> Product1/1, Product/2
  Trigonometric Function/1 -> Product1/2
  Product/1 -> Vector Concatenate2/1, Sum2/2
  Product1/1 -> Vector Concatenate2/2, Sum3/2
  Demux/3 -> Sum4/1
  Sum4/1 -> Trigonometric Function/1, Trigonometric Function1/1
  Constant3/1 -> Sum4/2
  Vector Concatenate/1 -> n3/1
  Vector Concatenate2/1 -> n1/1

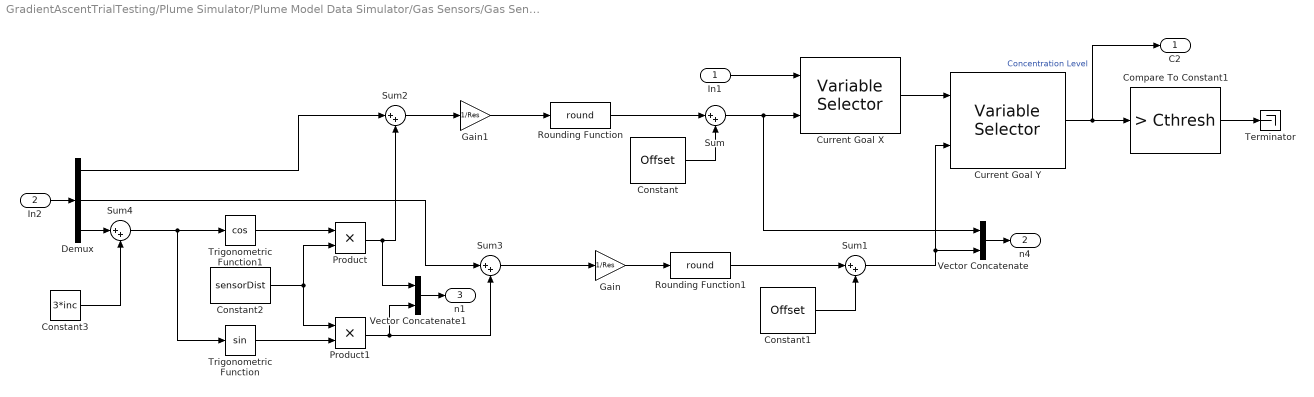
== system GradientAscentTrialTesting/Plume Simulator/Plume Model Data Simulator/Gas Sensors/Gas Sensor 4 ==
  In1 : Inport
  In2 : Inport  Port=2
  Compare To Constant1 : simulink/Logic and Bit Operations/Compare To Constant  relop=>  const=Cthresh  OutDataTypeStr=boolean
  Constant : Constant  Value=Offset
  Constant1 : Constant  Value=Offset
  Constant2 : Constant  Value=sensorDist
  Constant3 : Constant  Value=3*inc
  Current Goal X : dspindex/Variable Selector  NumInputs=1  rowsOrCols=Rows  IdxMode=Variable  Elements=[1 3]  ZerOneIdxMode=One-based  errmode=Clip Index  FillMode=off  FillValues=0
  Current Goal Y : dspindex/Variable Selector  NumInputs=1  rowsOrCols=Columns  IdxMode=Variable  Elements=[1 3]  ZerOneIdxMode=One-based  errmode=Clip Index  FillMode=off  FillValues=0
  Demux : Demux  Outputs=3
  Gain : Gain  Gain=1/Res
  Gain1 : Gain  Gain=1/Res
  Product : Product
  Product1 : Product
  Rounding Function : Rounding  Operator=round
  Rounding Function1 : Rounding  Operator=round
  Sum{,1..4} (5 alike) : Sum  Inputs=|++
  Terminator : Terminator
  Trigonometric Function : Trigonometry
  Trigonometric Function1 : Trigonometry  Operator=cos
  Vector Concatenate : Concatenate
  Vector Concatenate1 : Concatenate
  C2 : Outport
  n4 : Outport  Port=2
  n1 : Outport  Port=3
  wires:
  In1/1 -> Current Goal X/1
  Rounding Function/1 -> Sum/1
  Current Goal Y/1 -> C2/1, Compare To Constant1/1  "Concentration Level"
  Rounding Function1/1 -> Sum1/1
  Current Goal X/1 -> Current Goal Y/1
  Constant/1 -> Sum/2
  Compare To Constant1/1 -> Terminator/1
  Constant1/1 -> Sum1/2
  Sum/1 -> Vector Concatenate/1, Current Goal X/2
  Sum1/1 -> Vector Concatenate/2, Current Goal Y/2
  Gain1/1 -> Rounding Function/1
  Gain/1 -> Rounding Function1/1
  Sum2/1 -> Gain1/1
  Sum3/1 -> Gain/1
  In2/1 -> Demux/1
  Demux/1 -> Sum2/1
  Demux/2 -> Sum3/1
  Trigonometric Function1/1 -> Product/1
  Constant2/1 -> Product1/1, Product/2
  Trigonometric Function/1 -> Product1/2
  Product/1 -> Vector Concatenate1/1, Sum2/2
  Product1/1 -> Vector Concatenate1/2, Sum3/2
  Demux/3 -> Sum4/1
  Sum4/1 -> Trigonometric Function/1, Trigonometric Function1/1
  Constant3/1 -> Sum4/2
  Vector Concatenate/1 -> n4/1
  Vector Concatenate1/1 -> n1/1

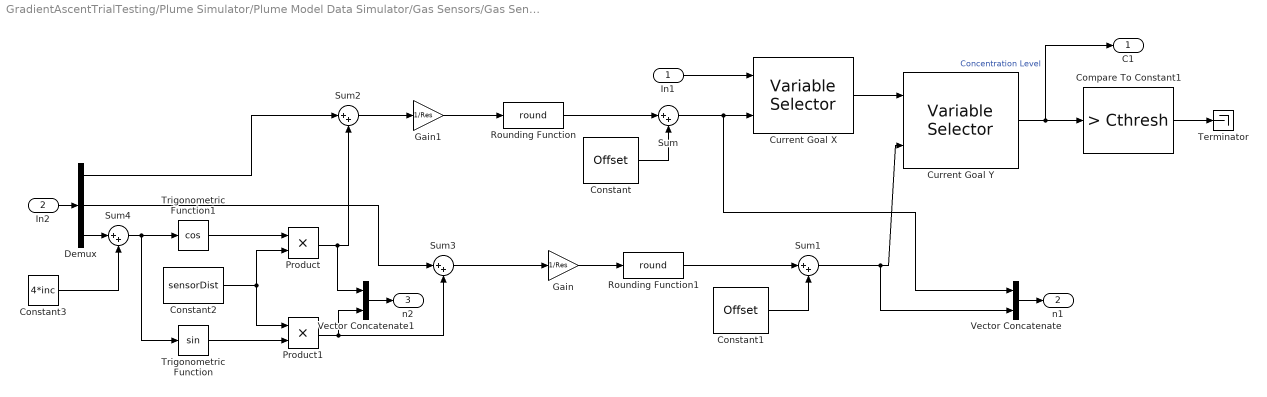
== system GradientAscentTrialTesting/Plume Simulator/Plume Model Data Simulator/Gas Sensors/Gas Sensor 5 ==
  In1 : Inport
  In2 : Inport  Port=2
  Compare To Constant1 : simulink/Logic and Bit Operations/Compare To Constant  relop=>  const=Cthresh  OutDataTypeStr=boolean
  Constant : Constant  Value=Offset
  Constant1 : Constant  Value=Offset
  Constant2 : Constant  Value=sensorDist
  Constant3 : Constant  Value=4*inc
  Current Goal X : dspindex/Variable Selector  NumInputs=1  rowsOrCols=Rows  IdxMode=Variable  Elements=[1 3]  ZerOneIdxMode=One-based  errmode=Clip Index  FillMode=off  FillValues=0
  Current Goal Y : dspindex/Variable Selector  NumInputs=1  rowsOrCols=Columns  IdxMode=Variable  Elements=[1 3]  ZerOneIdxMode=One-based  errmode=Clip Index  FillMode=off  FillValues=0
  Demux : Demux  Outputs=3
  Gain : Gain  Gain=1/Res
  Gain1 : Gain  Gain=1/Res
  Product : Product
  Product1 : Product
  Rounding Function : Rounding  Operator=round
  Rounding Function1 : Rounding  Operator=round
  Sum{,1..4} (5 alike) : Sum  Inputs=|++
  Terminator : Terminator
  Trigonometric Function : Trigonometry
  Trigonometric Function1 : Trigonometry  Operator=cos
  Vector Concatenate : Concatenate
  Vector Concatenate1 : Concatenate
  C1 : Outport
  n1 : Outport  Port=2
  n2 : Outport  Port=3
  wires:
  In1/1 -> Current Goal X/1
  Rounding Function/1 -> Sum/1
  Current Goal Y/1 -> C1/1, Compare To Constant1/1  "Concentration Level"
  Rounding Function1/1 -> Sum1/1
  Current Goal X/1 -> Current Goal Y/1
  Constant/1 -> Sum/2
  Compare To Constant1/1 -> Terminator/1
  Constant1/1 -> Sum1/2
  Sum/1 -> Vector Concatenate/1, Current Goal X/2
  Sum1/1 -> Vector Concatenate/2, Current Goal Y/2
  Gain1/1 -> Rounding Function/1
  Gain/1 -> Rounding Function1/1
  Sum2/1 -> Gain1/1
  Sum3/1 -> Gain/1
  In2/1 -> Demux/1
  Demux/1 -> Sum2/1
  Demux/2 -> Sum3/1
  Trigonometric Function1/1 -> Product/1
  Constant2/1 -> Product1/1, Product/2
  Trigonometric Function/1 -> Product1/2
  Product/1 -> Vector Concatenate1/1, Sum2/2
  Product1/1 -> Vector Concatenate1/2, Sum3/2
  Vector Concatenate/1 -> n1/1
  Demux/3 -> Sum4/1
  Sum4/1 -> Trigonometric Function/1, Trigonometric Function1/1
  Constant3/1 -> Sum4/2
  Vector Concatenate1/1 -> n2/1

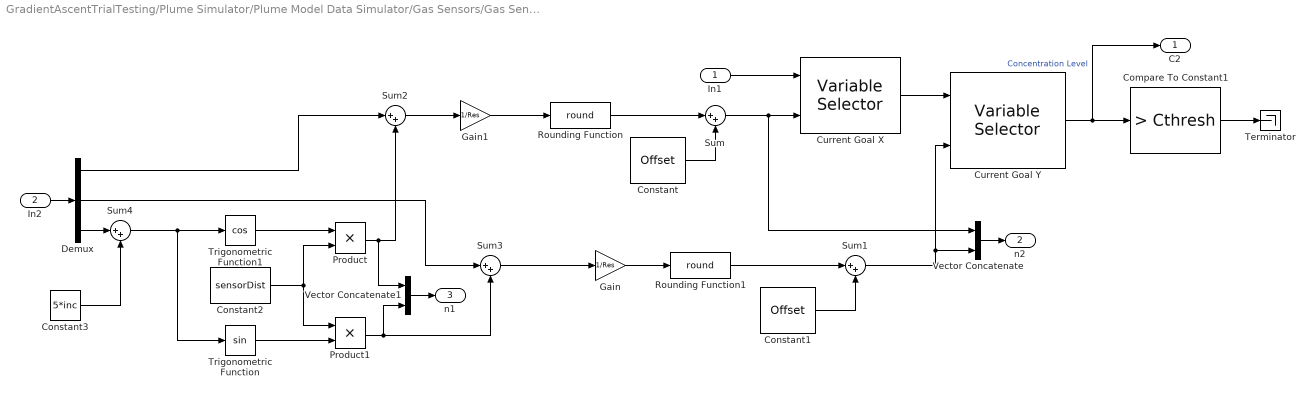
== system GradientAscentTrialTesting/Plume Simulator/Plume Model Data Simulator/Gas Sensors/Gas Sensor 6 ==
  In1 : Inport
  In2 : Inport  Port=2
  Compare To Constant1 : simulink/Logic and Bit Operations/Compare To Constant  relop=>  const=Cthresh  OutDataTypeStr=boolean
  Constant : Constant  Value=Offset
  Constant1 : Constant  Value=Offset
  Constant2 : Constant  Value=sensorDist
  Constant3 : Constant  Value=5*inc
  Current Goal X : dspindex/Variable Selector  NumInputs=1  rowsOrCols=Rows  IdxMode=Variable  Elements=[1 3]  ZerOneIdxMode=One-based  errmode=Clip Index  FillMode=off  FillValues=0
  Current Goal Y : dspindex/Variable Selector  NumInputs=1  rowsOrCols=Columns  IdxMode=Variable  Elements=[1 3]  ZerOneIdxMode=One-based  errmode=Clip Index  FillMode=off  FillValues=0
  Demux : Demux  Outputs=3
  Gain : Gain  Gain=1/Res
  Gain1 : Gain  Gain=1/Res
  Product : Product
  Product1 : Product
  Rounding Function : Rounding  Operator=round
  Rounding Function1 : Rounding  Operator=round
  Sum{,1..4} (5 alike) : Sum  Inputs=|++
  Terminator : Terminator
  Trigonometric Function : Trigonometry
  Trigonometric Function1 : Trigonometry  Operator=cos
  Vector Concatenate : Concatenate
  Vector Concatenate1 : Concatenate
  C2 : Outport
  n2 : Outport  Port=2
  n1 : Outport  Port=3
  wires:
  In1/1 -> Current Goal X/1
  Rounding Function/1 -> Sum/1
  Current Goal Y/1 -> C2/1, Compare To Constant1/1  "Concentration Level"
  Rounding Function1/1 -> Sum1/1
  Current Goal X/1 -> Current Goal Y/1
  Constant/1 -> Sum/2
  Compare To Constant1/1 -> Terminator/1
  Constant1/1 -> Sum1/2
  Sum/1 -> Vector Concatenate/1, Current Goal X/2
  Sum1/1 -> Vector Concatenate/2, Current Goal Y/2
  Gain1/1 -> Rounding Function/1
  Gain/1 -> Rounding Function1/1
  Sum2/1 -> Gain1/1
  Sum3/1 -> Gain/1
  In2/1 -> Demux/1
  Demux/1 -> Sum2/1
  Demux/2 -> Sum3/1
  Trigonometric Function1/1 -> Product/1
  Constant2/1 -> Product1/1, Product/2
  Trigonometric Function/1 -> Product1/2
  Product/1 -> Vector Concatenate1/1, Sum2/2
  Product1/1 -> Vector Concatenate1/2, Sum3/2
  Demux/3 -> Sum4/1
  Sum4/1 -> Trigonometric Function/1, Trigonometric Function1/1
  Constant3/1 -> Sum4/2
  Vector Concatenate/1 -> n2/1
  Vector Concatenate1/1 -> n1/1
